simulink model "PubIfDecisionTOS_MDL"  (R2020b)
settings: configuration reference "DspaceConfig" (kept outside this file)
PostLoadFcn:
  | if any(exist('dsrtsu_mdlpostloadfcn', 'file') ~= 0), dsrtsu_mdlpostloadfcn('Execute', bdroot); end
InitFcn:
  | , if any(exist('dsmpb_private', 'file') ~= 0), dsmpb_private('dsmpb_mdlclblib', 'Init', bdroot); end,
undefined symbols (not defined in the file or in its folder): C_TOS_ACCEgoRAxletoFbumplength_m, C_TOS_ACCTargetFront_Flag, C_TOS_AEBJAPedObjDxThre_Val, C_TOS_AEBJAPedObjDyThre_Val, C_TOS_AEBJATargetSize_Val, C_TOS_AEBJAVehObjDxThre_Val, C_TOS_AEBJAVehObjDyThre_Val, C_TOS_AEBJuncPedTargetSize_Val, C_TOS_AEBLatObjDxThre_Val, C_TOS_AEBLatPedDyThre_Val, C_TOS_AEBLatTargetSize_Val, C_TOS_AEBLongTargetInEgoFront_Flag, C_TOS_axAbsGround_Parameter, C_TOS_CameraConfirmedFlag, C_TOS_CNsubjWidth, C_TOS_CurrentLaneCoreMinWidth_Val, C_TOS_CutInProb_Val_Zero, C_TOS_CutOutProb_Val_Zero, C_TOS_D2R_Val, C_TOS_DefaultValueObjectToCenterLine_dy, C_TOS_EgoCarWidth_Val, C_TOS_EgoDxRefPoint_m, C_TOS_EgoRAxletoFbumplength_m, C_TOS_HalfWidthVehicle_Con, C_TOS_HWA_CurrentLaneFlag, C_TOS_HWA_LeftLaneFlag, C_TOS_HWA_MovingDir_Vaild, C_TOS_HWA_MovState_Vaild, C_TOS_HWA_RightLaneFlag, C_TOS_LaneLineCourseErrorFront, C_TOS_LaneLineCourseErrorRear, C_TOS_MotorbikeDefaultWidth_m, C_TOS_NumberOfEffectiveTargets, C_TOS_Obj_Age_Val, C_TOS_Objdx_Constraint_Val, C_TOS_ObjectDefaultWidth_m, C_TOS_ObjInCurrentLane_Val, C_TOS_ObjInCurrentLaneValid, C_TOS_ObjInLeftLaneValid, C_TOS_ObjInRightLaneValid, C_TOS_ObjNotInCurrentLane_Val, C_TOS_ObjNotREElementType, C_TOS_ObjPredictDis_dy_ConstantVal_Zeros, C_TOS_ObjToCenterLine_ConstantVal_Zeros, C_TOS_OFMObjIDInvilad_Val, C_TOS_PIL_LatDisCons_Val_zero, C_TOS_PIL_ObjectCutInFlag_b, C_TOS_PIL_ObjectCutOutFlag_b, C_TOS_PIL_ObjLaneProb_al_Val, C_TOS_PP_ObjFusType_FC_Confirm_b, C_TOS_PP_ObjFusType_FC_FR_Confirm_b, C_TOS_PP_ObjFusType_FR_Confirm_b, C_TOS_RE_80BoolDefault_Val, C_TOS_RE_80Single181Default_Val, C_TOS_RE_80Single255Default_Val, C_TOS_RE_80Uint8Default_Val, C_TOS_RE_D2R, C_TOS_RE_D_180_Val, C_TOS_RE_InvalidObjectID_Val, C_TOS_RE_InvalidTargetChainDir_Val ... (+142)
libraries: simulink x1650, TOS_LIB x361, canfdmsglib x14
(part 20 of 69)

== system PubIfDecisionTOS_MDL/TOS_20201112/TOS_2012080320/TOS/ACC/TOS_ACCRightLane/ACC_Object_PreConfirm/ACC_Object_PreConfirm ==
  PP_ObjFusType_FC_FR_Confirm : Inport  Partition=on  PartitionDimension=1  PartitionWidth=1  PartitionOffset=0
  PP_ObjFusType_FR_Confirm : Inport  Port=2  Partition=on  PartitionDimension=1  PartitionWidth=1  PartitionOffset=0
  PP_ObjFusType_FC_Confirm : Inport  Port=3  Partition=on  PartitionDimension=1  PartitionWidth=1  PartitionOffset=0
  Object_ID : Inport  Port=4  OutDataTypeStr=uint8  Partition=on  PartitionDimension=1  PartitionWidth=1  PartitionOffset=0
  Obj_MovingState : Inport  Port=5  Partition=on  PartitionDimension=1  PartitionWidth=1  PartitionOffset=0
  Obj_Dx : Inport  Port=6  Partition=on  PartitionDimension=1  PartitionWidth=1  PartitionOffset=0
  Object_ObstacleProb : Inport  Port=7  Partition=on  PartitionDimension=1  PartitionWidth=1  PartitionOffset=0
  Object_DY : Inport  Port=8  Partition=on  PartitionDimension=1  PartitionWidth=1  PartitionOffset=0
  Object_ObjType : Inport  Port=9  Partition=on  PartitionDimension=1  PartitionWidth=1  PartitionOffset=0
  ACC_Target_ID_K1 : Inport  Port=10
  ACC_Target_Dx_K1 : Inport  Port=11
  ACC_Object_PreConfirm : Subsystem
  ACC_Object_PreConfirmDefault : Subsystem  TreatAsAtomicUnit=on
  Compare To Constant : simulink/Logic and Bit Operations/Compare To Constant  relop===  const=C_TOS_OFMObjIDInvilad_Val  OutDataTypeStr=boolean
      settings: AttributesFormatString=C_TOS_OFMObjIDInvilad_Val = 0
  For Each : ForEach  DisableCoverage=on
  If : If  IfExpression=u1 ~= 0
  Merge{,1,3..5} (5 alike) : Merge
  TOS_ACC_TargetPre_Confirm_FiltFlag : Outport  ConcatenationDimension=1
  TOS_ACC_TargetPre_FusionTypeFlag_ObserVale : Outport  Port=2  ConcatenationDimension=1
  TOS_ACC_TargetPre_PassedbyTarget_ObserVale : Outport  Port=3  ConcatenationDimension=1
  TOS_ACC_TargetPre_ObjType_ObserVale : Outport  Port=4  ConcatenationDimension=1
  TOS_ACC_DyConfirm_ObserVale : Outport  Port=5  ConcatenationDimension=1
  wires:
  Merge4/1 -> TOS_ACC_DyConfirm_ObserVale/1
  Merge3/1 -> TOS_ACC_TargetPre_ObjType_ObserVale/1
  Merge1/1 -> TOS_ACC_TargetPre_PassedbyTarget_ObserVale/1
  Merge5/1 -> TOS_ACC_TargetPre_FusionTypeFlag_ObserVale/1
  Merge/1 -> TOS_ACC_TargetPre_Confirm_FiltFlag/1
  ACC_Object_PreConfirmDefault/5(TOS_ACC_DyConfirm_ObserVale) -> Merge4/1
  ACC_Object_PreConfirmDefault/4(TOS_ACC_TargetPre_ObjType_ObserVale) -> Merge3/1
  ACC_Object_PreConfirmDefault/3(TOS_ACC_TargetPre_PassedbyTarget_ObserVale) -> Merge1/1
  ACC_Object_PreConfirmDefault/2(TOS_ACC_TargetPre_FusionTypeFlag_ObserVale) -> Merge5/1
  ACC_Object_PreConfirmDefault/1(TOS_ACC_TargetPre_Confirm_FiltFlag) -> Merge/1
  ACC_Object_PreConfirm/5(TOS_ACC_DyConfirm_ObserVale) -> Merge4/2
  ACC_Object_PreConfirm/4(TOS_ACC_TargetPre_ObjType_ObserVale) -> Merge3/2
  ACC_Object_PreConfirm/3(TOS_ACC_TargetPre_PassedbyTarget_ObserVale) -> Merge1/2
  ACC_Object_PreConfirm/2(TOS_ACC_TargetPre_FusionTypeFlag_ObserVale) -> Merge5/2
  ACC_Object_PreConfirm/1(TOS_ACC_TargetPre_Confirm_FiltFlag) -> Merge/2
  Object_ObjType/1 -> ACC_Object_PreConfirm/9(Object_ObjType)
  [Object_ID] -> ACC_Object_PreConfirm/1(Object_ID)
  ACC_Target_Dx_K1/1 -> ACC_Object_PreConfirm/11(ACC_Target_Dx_K1)
  ACC_Target_ID_K1/1 -> ACC_Object_PreConfirm/10(ACC_Target_ID_K1)
  Object_DY/1 -> ACC_Object_PreConfirm/8(Object_DY)
  Object_ObstacleProb/1 -> ACC_Object_PreConfirm/7(Object_ObstacleProb)
  Obj_Dx/1 -> ACC_Object_PreConfirm/6(Obj_Dx)
  Obj_MovingState/1 -> ACC_Object_PreConfirm/5(Obj_MovingState)
  PP_ObjFusType_FC_Confirm/1 -> ACC_Object_PreConfirm/4(PP_ObjFusType_FC_Confirm)
  If/2 -> ACC_Object_PreConfirm/Action
  If/1 -> ACC_Object_PreConfirmDefault/Action
  Object_ID/1 -> Compare To Constant/1, [Object_ID]
  Compare To Constant/1 -> If/1
  PP_ObjFusType_FR_Confirm/1 -> ACC_Object_PreConfirm/3(PP_ObjFusType_FR_Confirm)
  PP_ObjFusType_FC_FR_Confirm/1 -> ACC_Object_PreConfirm/2(PP_ObjFusType_FC_FR_Confirm)

== system PubIfDecisionTOS_MDL/TOS_20201112/TOS_2012080320/TOS/AEB/TOS_AEBJunct1105/AEBJunc_Object_Condition/AEBJA_TargetCondition ==
  Object_ID : Inport  OutDataTypeStr=uint8  Partition=on  PartitionDimension=1  PartitionWidth=1  PartitionOffset=0
  PP_ObjFusType_FC_FR_Confirm : Inport  Port=2  Partition=on  PartitionDimension=1  PartitionWidth=1  PartitionOffset=0
  PP_ObjFusType_FR_Confirm : Inport  Port=3  Partition=on  PartitionDimension=1  PartitionWidth=1  PartitionOffset=0
  ObjectType : Inport  Port=4  Partition=on  PartitionDimension=1  PartitionWidth=1  PartitionOffset=0
  Object_Dx : Inport  Port=5  Partition=on  PartitionDimension=1  PartitionWidth=1  PartitionOffset=0
  Object_Dy : Inport  Port=6  Partition=on  PartitionDimension=1  PartitionWidth=1  PartitionOffset=0
  PP_ObjMovingDirSignalProcessing : Inport  Port=7  Partition=on  PartitionDimension=1  PartitionWidth=1  PartitionOffset=0
  Object_HeadingAngle : Inport  Port=8  Partition=on  PartitionDimension=1  PartitionWidth=1  PartitionOffset=0
  Object_VX : Inport  Port=9  Partition=on  PartitionDimension=1  PartitionWidth=1  PartitionOffset=0
  Object_VY : Inport  Port=10  Partition=on  PartitionDimension=1  PartitionWidth=1  PartitionOffset=0
  VIE_EgoVelocity : Inport  Port=11
  psiDtOpt : Inport  Port=12
  axvRefMs2 : Inport  Port=13
  Object_MovingState : Inport  Port=14  Partition=on  PartitionDimension=1  PartitionWidth=1  PartitionOffset=0
  AEBJunc_Target_ObjectID_K1 : Inport  Port=15
  AEBJunc_Target_ObjectType_K1 : Inport  Port=16
  Compare To Constant : simulink/Logic and Bit Operations/Compare To Constant  relop===  const=C_TOS_OFMObjIDInvilad_Val  OutDataTypeStr=boolean
      settings: AttributesFormatString=C_TOS_OFMObjIDInvilad_Val = 0
  For Each : ForEach  DisableCoverage=on
  If : If  IfExpression=u1 ~= 0
  Merge{,1..10} (11 alike) : Merge
  TOS_AEBJunc_TargetsCondition : Subsystem
  TOS_AEBJunc_TargetsConditionDefault : Subsystem  TreatAsAtomicUnit=on
  TOS_AEBJunc_PedTargets_Dx : Outport  ConcatenationDimension=1
  TOS_AEBJunc_VehTargets_Dx : Outport  Port=2  ConcatenationDimension=1
  AEBJunc_PedTargetFusionType_observal : Outport  Port=3  ConcatenationDimension=1
  AEBJunc_PedTargetObjectType_observal : Outport  Port=4  ConcatenationDimension=1
  AEBJunc_PedTargetDXDY_observal : Outport  Port=5  ConcatenationDimension=1
  AEBJunc_PedTargetMovDir_observal : Outport  Port=6  ConcatenationDimension=1
  AEBJunc_VehTargetFusionType_observal : Outport  Port=7  ConcatenationDimension=1
  AEBJunc_VehTargetObjectType_observal : Outport  Port=8  ConcatenationDimension=1
  AEBJunc_VehTargetDXDY_observal : Outport  Port=9  ConcatenationDimension=1
  AEBJunc_VehTargetMovDir_observal : Outport  Port=10  ConcatenationDimension=1
  AEBJunc_VehTargetMovState_observal : Outport  Port=11  ConcatenationDimension=1
  wires:
  PP_ObjFusType_FC_FR_Confirm/1 -> TOS_AEBJunc_TargetsCondition/2(PP_ObjFusType_FC_FR_Confirm)
  PP_ObjFusType_FR_Confirm/1 -> TOS_AEBJunc_TargetsCondition/3(PP_ObjFusType_FR_Confirm)
  Object_VY/1 -> TOS_AEBJunc_TargetsCondition/10(Object_VY)
  VIE_EgoVelocity/1 -> TOS_AEBJunc_TargetsCondition/11(VIE_EgoVelocity)
  Object_VX/1 -> TOS_AEBJunc_TargetsCondition/9(Object_VX)
  PP_ObjMovingDirSignalProcessing/1 -> TOS_AEBJunc_TargetsCondition/7(PP_ObjMovingDirSignalProcessing)
  Object_HeadingAngle/1 -> TOS_AEBJunc_TargetsCondition/8(Object_HeadingAngle)
  ObjectType/1 -> TOS_AEBJunc_TargetsCondition/4(ObjectType)
  TOS_AEBJunc_TargetsConditionDefault/1(TOS_AEBJunc_PedTargetsDx) -> Merge/1
  If/2 -> TOS_AEBJunc_TargetsCondition/Action
  If/1 -> TOS_AEBJunc_TargetsConditionDefault/Action
  Object_ID/1 -> Compare To Constant/1, [Object_ID]
  Compare To Constant/1 -> If/1
  TOS_AEBJunc_TargetsCondition/1(TOS_AEBJunc_PedTargetsDx) -> Merge/2
  Object_Dy/1 -> TOS_AEBJunc_TargetsCondition/6(Object_Dy)
  Object_Dx/1 -> TOS_AEBJunc_TargetsCondition/5(Object_Dx)
  Merge/1 -> TOS_AEBJunc_PedTargets_Dx/1
  TOS_AEBJunc_TargetsCondition/3(AEBJunc_PedTargetFusionType_observal) -> Merge1/2
  TOS_AEBJunc_TargetsConditionDefault/3(AEBJunc_PedTargetFusionType_observal) -> Merge1/1
  TOS_AEBJunc_TargetsConditionDefault/4(AEBJunc_PedTargetObjectType_observal) -> Merge2/1
  TOS_AEBJunc_TargetsCondition/4(AEBJunc_PedTargetObjectType_observal) -> Merge2/2
  TOS_AEBJunc_TargetsCondition/5(AEBJunc_PedTargetDXDY_observal) -> Merge3/2
  TOS_AEBJunc_TargetsConditionDefault/5(AEBJunc_PedTargetDXDY_observal) -> Merge3/1
  TOS_AEBJunc_TargetsConditionDefault/6(AEBJunc_PedTargetMovDir_observal) -> Merge4/1
  TOS_AEBJunc_TargetsCondition/6(AEBJunc_PedTargetMovDir_observal) -> Merge4/2
  Merge1/1 -> AEBJunc_PedTargetFusionType_observal/1
  Merge2/1 -> AEBJunc_PedTargetObjectType_observal/1
  Merge3/1 -> AEBJunc_PedTargetDXDY_observal/1
  Merge4/1 -> AEBJunc_PedTargetMovDir_observal/1
  [Object_ID] -> TOS_AEBJunc_TargetsCondition/1(Object_ID)  "Object_ID"
  AEBJunc_Target_ObjectID_K1/1 -> TOS_AEBJunc_TargetsCondition/15(AEBJunc_Target_ObjectID_K1)
  psiDtOpt/1 -> TOS_AEBJunc_TargetsCondition/12(psiDtOpt)
  axvRefMs2/1 -> TOS_AEBJunc_TargetsCondition/13(axvRefMs2)  "axvRefMs2"
  AEBJunc_Target_ObjectType_K1/1 -> TOS_AEBJunc_TargetsCondition/16(AEBJunc_Target_ObjectType_K1)  "AEBJunc_Target_ObjectType_K1"
  Merge5/1 -> TOS_AEBJunc_VehTargets_Dx/1
  TOS_AEBJunc_TargetsCondition/2(TOS_AEBJunc_VehTargetsDx) -> Merge5/2
  TOS_AEBJunc_TargetsConditionDefault/2(TOS_AEBJunc_VehTargetsDx) -> Merge5/1
  Merge9/1 -> AEBJunc_VehTargetMovDir_observal/1
  Merge8/1 -> AEBJunc_VehTargetDXDY_observal/1
  Merge7/1 -> AEBJunc_VehTargetObjectType_observal/1
  Merge6/1 -> AEBJunc_VehTargetFusionType_observal/1
  TOS_AEBJunc_TargetsCondition/10(AEBJunc_VehTargetMovDir_observal) -> Merge9/2
  TOS_AEBJunc_TargetsConditionDefault/10(AEBJunc_VehTargetMovDir_observal) -> Merge9/1
  TOS_AEBJunc_TargetsConditionDefault/9(AEBJunc_VehTargetDXDY_observal) -> Merge8/1
  TOS_AEBJunc_TargetsCondition/9(AEBJunc_VehTargetDXDY_observal) -> Merge8/2
  TOS_AEBJunc_TargetsCondition/8(AEBJunc_VehTargetObjectType_observal) -> Merge7/2
  TOS_AEBJunc_TargetsConditionDefault/8(AEBJunc_VehTargetObjectType_observal) -> Merge7/1
  TOS_AEBJunc_TargetsConditionDefault/7(AEBJunc_VehTargetFusionType_observal) -> Merge6/1
  TOS_AEBJunc_TargetsCondition/7(AEBJunc_VehTargetFusionType_observal) -> Merge6/2
  Object_MovingState/1 -> TOS_AEBJunc_TargetsCondition/14(Object_MovingState)  "Object_MovingState"
  TOS_AEBJunc_TargetsConditionDefault/11(AEBJunc_VehTargetMovState_observal) -> Merge10/1
  TOS_AEBJunc_TargetsCondition/11(AEBJunc_VehTargetMovState_observal) -> Merge10/2
  Merge10/1 -> AEBJunc_VehTargetMovState_observal/1

== system PubIfDecisionTOS_MDL/TOS_20201112/TOS_2012080320/TOS/AEB/TOS_AEBJunct1105/AEBJunc_Object_Condition1/AEBJA_TargetCondition ==
  Object_ID : Inport  OutDataTypeStr=uint8  Partition=on  PartitionDimension=1  PartitionWidth=1  PartitionOffset=0
  PP_ObjFusType_FC_FR_Confirm : Inport  Port=2  Partition=on  PartitionDimension=1  PartitionWidth=1  PartitionOffset=0
  PP_ObjFusType_FR_Confirm : Inport  Port=3  Partition=on  PartitionDimension=1  PartitionWidth=1  PartitionOffset=0
  ObjectType : Inport  Port=4  Partition=on  PartitionDimension=1  PartitionWidth=1  PartitionOffset=0
  Object_Dx : Inport  Port=5  Partition=on  PartitionDimension=1  PartitionWidth=1  PartitionOffset=0
  Object_Dy : Inport  Port=6  Partition=on  PartitionDimension=1  PartitionWidth=1  PartitionOffset=0
  PP_ObjMovingDirSignalProcessing : Inport  Port=7  Partition=on  PartitionDimension=1  PartitionWidth=1  PartitionOffset=0
  Object_HeadingAngle : Inport  Port=8  Partition=on  PartitionDimension=1  PartitionWidth=1  PartitionOffset=0
  Object_VX : Inport  Port=9  Partition=on  PartitionDimension=1  PartitionWidth=1  PartitionOffset=0
  Object_VY : Inport  Port=10  Partition=on  PartitionDimension=1  PartitionWidth=1  PartitionOffset=0
  VIE_EgoVelocity : Inport  Port=11
  psiDtOpt : Inport  Port=12
  axvRefMs2 : Inport  Port=13
  Object_MovingState : Inport  Port=14  Partition=on  PartitionDimension=1  PartitionWidth=1  PartitionOffset=0
  AEBJunc_Target_ObjectID_K1 : Inport  Port=15
  AEBJunc_Target_ObjectType_K1 : Inport  Port=16
  Compare To Constant : simulink/Logic and Bit Operations/Compare To Constant  relop===  const=C_TOS_OFMObjIDInvilad_Val  OutDataTypeStr=boolean
      settings: AttributesFormatString=C_TOS_OFMObjIDInvilad_Val = 0
  For Each : ForEach  DisableCoverage=on
  If : If  IfExpression=u1 ~= 0
  Merge{,1..10} (11 alike) : Merge
  TOS_AEBJunc_TargetsCondition : Subsystem
  TOS_AEBJunc_TargetsConditionDefault : Subsystem  TreatAsAtomicUnit=on
  TOS_AEBJunc_PedTargets_Dx : Outport  ConcatenationDimension=1
  TOS_AEBJunc_VehTargets_Dx : Outport  Port=2  ConcatenationDimension=1
  AEBJunc_PedTargetFusionType_observal : Outport  Port=3  ConcatenationDimension=1
  AEBJunc_PedTargetObjectType_observal : Outport  Port=4  ConcatenationDimension=1
  AEBJunc_PedTargetDXDY_observal : Outport  Port=5  ConcatenationDimension=1
  AEBJunc_PedTargetMovDir_observal : Outport  Port=6  ConcatenationDimension=1
  AEBJunc_VehTargetFusionType_observal : Outport  Port=7  ConcatenationDimension=1
  AEBJunc_VehTargetObjectType_observal : Outport  Port=8  ConcatenationDimension=1
  AEBJunc_VehTargetDXDY_observal : Outport  Port=9  ConcatenationDimension=1
  AEBJunc_VehTargetMovDir_observal : Outport  Port=10  ConcatenationDimension=1
  AEBJunc_VehTargetMovState_observal : Outport  Port=11  ConcatenationDimension=1
  wires:
  Merge10/1 -> AEBJunc_VehTargetMovState_observal/1
  TOS_AEBJunc_TargetsCondition/11(AEBJunc_VehTargetMovState_observal) -> Merge10/2
  TOS_AEBJunc_TargetsConditionDefault/11(AEBJunc_VehTargetMovState_observal) -> Merge10/1
  Object_MovingState/1 -> TOS_AEBJunc_TargetsCondition/14(Object_MovingState)  "Object_MovingState"
  TOS_AEBJunc_TargetsCondition/7(AEBJunc_VehTargetFusionType_observal) -> Merge6/2
  TOS_AEBJunc_TargetsConditionDefault/7(AEBJunc_VehTargetFusionType_observal) -> Merge6/1
  TOS_AEBJunc_TargetsConditionDefault/8(AEBJunc_VehTargetObjectType_observal) -> Merge7/1
  TOS_AEBJunc_TargetsCondition/8(AEBJunc_VehTargetObjectType_observal) -> Merge7/2
  TOS_AEBJunc_TargetsCondition/9(AEBJunc_VehTargetDXDY_observal) -> Merge8/2
  TOS_AEBJunc_TargetsConditionDefault/9(AEBJunc_VehTargetDXDY_observal) -> Merge8/1
  TOS_AEBJunc_TargetsConditionDefault/10(AEBJunc_VehTargetMovDir_observal) -> Merge9/1
  TOS_AEBJunc_TargetsCondition/10(AEBJunc_VehTargetMovDir_observal) -> Merge9/2
  Merge6/1 -> AEBJunc_VehTargetFusionType_observal/1
  Merge7/1 -> AEBJunc_VehTargetObjectType_observal/1
  Merge8/1 -> AEBJunc_VehTargetDXDY_observal/1
  Merge9/1 -> AEBJunc_VehTargetMovDir_observal/1
  TOS_AEBJunc_TargetsConditionDefault/2(TOS_AEBJunc_VehTargetsDx) -> Merge5/1
  TOS_AEBJunc_TargetsCondition/2(TOS_AEBJunc_VehTargetsDx) -> Merge5/2
  Merge5/1 -> TOS_AEBJunc_VehTargets_Dx/1
  AEBJunc_Target_ObjectType_K1/1 -> TOS_AEBJunc_TargetsCondition/16(AEBJunc_Target_ObjectType_K1)  "AEBJunc_Target_ObjectType_K1"
  axvRefMs2/1 -> TOS_AEBJunc_TargetsCondition/13(axvRefMs2)  "axvRefMs2"
  psiDtOpt/1 -> TOS_AEBJunc_TargetsCondition/12(psiDtOpt)
  AEBJunc_Target_ObjectID_K1/1 -> TOS_AEBJunc_TargetsCondition/15(AEBJunc_Target_ObjectID_K1)
  [Object_ID] -> TOS_AEBJunc_TargetsCondition/1(Object_ID)  "Object_ID"
  Merge4/1 -> AEBJunc_PedTargetMovDir_observal/1
  Merge3/1 -> AEBJunc_PedTargetDXDY_observal/1
  Merge2/1 -> AEBJunc_PedTargetObjectType_observal/1
  Merge1/1 -> AEBJunc_PedTargetFusionType_observal/1
  TOS_AEBJunc_TargetsCondition/6(AEBJunc_PedTargetMovDir_observal) -> Merge4/2
  TOS_AEBJunc_TargetsConditionDefault/6(AEBJunc_PedTargetMovDir_observal) -> Merge4/1
  TOS_AEBJunc_TargetsConditionDefault/5(AEBJunc_PedTargetDXDY_observal) -> Merge3/1
  TOS_AEBJunc_TargetsCondition/5(AEBJunc_PedTargetDXDY_observal) -> Merge3/2
  TOS_AEBJunc_TargetsCondition/4(AEBJunc_PedTargetObjectType_observal) -> Merge2/2
  TOS_AEBJunc_TargetsConditionDefault/4(AEBJunc_PedTargetObjectType_observal) -> Merge2/1
  TOS_AEBJunc_TargetsConditionDefault/3(AEBJunc_PedTargetFusionType_observal) -> Merge1/1
  TOS_AEBJunc_TargetsCondition/3(AEBJunc_PedTargetFusionType_observal) -> Merge1/2
  Merge/1 -> TOS_AEBJunc_PedTargets_Dx/1
  Object_Dx/1 -> TOS_AEBJunc_TargetsCondition/5(Object_Dx)
  Object_Dy/1 -> TOS_AEBJunc_TargetsCondition/6(Object_Dy)
  TOS_AEBJunc_TargetsCondition/1(TOS_AEBJunc_PedTargetsDx) -> Merge/2
  Compare To Constant/1 -> If/1
  Object_ID/1 -> [Object_ID], Compare To Constant/1
  If/1 -> TOS_AEBJunc_TargetsConditionDefault/Action
  If/2 -> TOS_AEBJunc_TargetsCondition/Action
  TOS_AEBJunc_TargetsConditionDefault/1(TOS_AEBJunc_PedTargetsDx) -> Merge/1
  ObjectType/1 -> TOS_AEBJunc_TargetsCondition/4(ObjectType)
  Object_HeadingAngle/1 -> TOS_AEBJunc_TargetsCondition/8(Object_HeadingAngle)
  PP_ObjMovingDirSignalProcessing/1 -> TOS_AEBJunc_TargetsCondition/7(PP_ObjMovingDirSignalProcessing)
  Object_VX/1 -> TOS_AEBJunc_TargetsCondition/9(Object_VX)
  VIE_EgoVelocity/1 -> TOS_AEBJunc_TargetsCondition/11(VIE_EgoVelocity)
  Object_VY/1 -> TOS_AEBJunc_TargetsCondition/10(Object_VY)
  PP_ObjFusType_FR_Confirm/1 -> TOS_AEBJunc_TargetsCondition/3(PP_ObjFusType_FR_Confirm)
  PP_ObjFusType_FC_FR_Confirm/1 -> TOS_AEBJunc_TargetsCondition/2(PP_ObjFusType_FC_FR_Confirm)

== system PubIfDecisionTOS_MDL/TOS_20201112/TOS_2012080320/TOS/AEB/TOS_AEBJunct1105/AEBJunctionTargetInfor/AEBJuncTargetObjectType ==
  OFM_SignalVerification : Inport
  AEBJunc_Target_ObjectID_K1 : Inport  Port=2
  AEBJunc_Target_ObjectType_K1 : Inport  Port=3
  TOS_AEBJuncTrg_Index : Inport  Port=4  OutDataTypeStr=uint8  Partition=on  PartitionDimension=1  PartitionWidth=1  PartitionOffset=0
  AEBJuncTargetObjectType : Subsystem  TreatAsAtomicUnit=on
  AEBJuncTargetObjectTypeDefault : Subsystem  TreatAsAtomicUnit=on
  Compare To Constant1 : simulink/Logic and Bit Operations/Compare To Constant  relop===  const=C_TOS_OFMObjIDInvilad_Val  OutDataTypeStr=boolean
      settings: AttributesFormatString=C_TOS_OFMObjIDInvilad_Val = 0
  For Each : ForEach  DisableCoverage=on
  If : If  IfExpression=u1
  Merge : Merge
  TOS_AEBJuncTargetObjectType : Outport  ConcatenationDimension=1
  wires:
  Merge/1 -> TOS_AEBJuncTargetObjectType/1
  AEBJuncTargetObjectTypeDefault/1(TOS_AEBJuncTargetObjectType) -> Merge/1
  AEBJuncTargetObjectType/1(AEBLat_TargetObjectType) -> Merge/2
  If/2 -> AEBJuncTargetObjectType/Action
  If/1 -> AEBJuncTargetObjectTypeDefault/Action
  OFM_SignalVerification/1 -> AEBJuncTargetObjectType/2(OFM_SignalVerification)
  Compare To Constant1/1 -> If/1
  TOS_AEBJuncTrg_Index/1 -> AEBJuncTargetObjectType/1(TOS_AEBJuncTrg_Index), Compare To Constant1/1
  AEBJunc_Target_ObjectID_K1/1 -> AEBJuncTargetObjectType/3(AEBJunc_Target_ObjectID_K1)  "AEBJunc_Target_ObjectID_K1"
  AEBJunc_Target_ObjectType_K1/1 -> AEBJuncTargetObjectType/4(AEBJunc_Target_ObjectType_K1)  "AEBJunc_Target_ObjectType_K1"

== system PubIfDecisionTOS_MDL/TOS_20201112/TOS_2012080320/TOS/AEB/TOS_AEBJunct_20201208/AEBJunc_Object_Condition/AEBJA_TargetCondition ==
  Object_ID : Inport  OutDataTypeStr=uint8  Partition=on  PartitionDimension=1  PartitionWidth=1  PartitionOffset=0
  PP_ObjFusType_FC_FR_Confirm : Inport  Port=2  Partition=on  PartitionDimension=1  PartitionWidth=1  PartitionOffset=0
  PP_ObjFusType_FR_Confirm : Inport  Port=3  Partition=on  PartitionDimension=1  PartitionWidth=1  PartitionOffset=0
  ObjectType : Inport  Port=4  Partition=on  PartitionDimension=1  PartitionWidth=1  PartitionOffset=0
  Object_Dx : Inport  Port=5  Partition=on  PartitionDimension=1  PartitionWidth=1  PartitionOffset=0
  Object_Dy : Inport  Port=6  Partition=on  PartitionDimension=1  PartitionWidth=1  PartitionOffset=0
  PP_ObjMovingDirSignalProcessing : Inport  Port=7  Partition=on  PartitionDimension=1  PartitionWidth=1  PartitionOffset=0
  Object_HeadingAngle : Inport  Port=8  Partition=on  PartitionDimension=1  PartitionWidth=1  PartitionOffset=0
  Object_VX : Inport  Port=9  Partition=on  PartitionDimension=1  PartitionWidth=1  PartitionOffset=0
  Object_VY : Inport  Port=10  Partition=on  PartitionDimension=1  PartitionWidth=1  PartitionOffset=0
  VIE_EgoVelocity : Inport  Port=11
  psiDtOpt : Inport  Port=12
  axvRefMs2 : Inport  Port=13
  Object_MovingState : Inport  Port=14  Partition=on  PartitionDimension=1  PartitionWidth=1  PartitionOffset=0
  AEBJunc_Target_ObjectID_K1 : Inport  Port=15
  AEBJunc_Target_ObjectType_K1 : Inport  Port=16
  Compare To Constant : simulink/Logic and Bit Operations/Compare To Constant  relop===  const=C_TOS_OFMObjIDInvilad_Val  OutDataTypeStr=boolean
      settings: AttributesFormatString=C_TOS_OFMObjIDInvilad_Val = 0
  For Each : ForEach  DisableCoverage=on
  If : If  IfExpression=u1 ~= 0
  Merge{,1..10} (11 alike) : Merge
  TOS_AEBJunc_TargetsCondition : Subsystem
  TOS_AEBJunc_TargetsConditionDefault : Subsystem  TreatAsAtomicUnit=on
  TOS_AEBJunc_PedTargets_Dx : Outport  ConcatenationDimension=1
  TOS_AEBJunc_VehTargets_Dx : Outport  Port=2  ConcatenationDimension=1
  AEBJunc_PedTargetFusionType_observal : Outport  Port=3  ConcatenationDimension=1
  AEBJunc_PedTargetObjectType_observal : Outport  Port=4  ConcatenationDimension=1
  AEBJunc_PedTargetDXDY_observal : Outport  Port=5  ConcatenationDimension=1
  AEBJunc_PedTargetMovDir_observal : Outport  Port=6  ConcatenationDimension=1
  AEBJunc_VehTargetFusionType_observal : Outport  Port=7  ConcatenationDimension=1
  AEBJunc_VehTargetObjectType_observal : Outport  Port=8  ConcatenationDimension=1
  AEBJunc_VehTargetDXDY_observal : Outport  Port=9  ConcatenationDimension=1
  AEBJunc_VehTargetMovDir_observal : Outport  Port=10  ConcatenationDimension=1
  AEBJunc_VehTargetMovState_observal : Outport  Port=11  ConcatenationDimension=1
  wires:
  PP_ObjFusType_FC_FR_Confirm/1 -> TOS_AEBJunc_TargetsCondition/2(PP_ObjFusType_FC_FR_Confirm)
  PP_ObjFusType_FR_Confirm/1 -> TOS_AEBJunc_TargetsCondition/3(PP_ObjFusType_FR_Confirm)
  Object_VY/1 -> TOS_AEBJunc_TargetsCondition/10(Object_VY)
  VIE_EgoVelocity/1 -> TOS_AEBJunc_TargetsCondition/11(VIE_EgoVelocity)
  Object_VX/1 -> TOS_AEBJunc_TargetsCondition/9(Object_VX)
  PP_ObjMovingDirSignalProcessing/1 -> TOS_AEBJunc_TargetsCondition/7(PP_ObjMovingDirSignalProcessing)
  Object_HeadingAngle/1 -> TOS_AEBJunc_TargetsCondition/8(Object_HeadingAngle)
  ObjectType/1 -> TOS_AEBJunc_TargetsCondition/4(ObjectType)
  TOS_AEBJunc_TargetsConditionDefault/1(TOS_AEBJunc_PedTargetsDx) -> Merge/1
  If/2 -> TOS_AEBJunc_TargetsCondition/Action
  If/1 -> TOS_AEBJunc_TargetsConditionDefault/Action
  Object_ID/1 -> Compare To Constant/1, [Object_ID]
  Compare To Constant/1 -> If/1
  TOS_AEBJunc_TargetsCondition/1(TOS_AEBJunc_PedTargetsDx) -> Merge/2
  Object_Dy/1 -> TOS_AEBJunc_TargetsCondition/6(Object_Dy)
  Object_Dx/1 -> TOS_AEBJunc_TargetsCondition/5(Object_Dx)
  Merge/1 -> TOS_AEBJunc_PedTargets_Dx/1
  TOS_AEBJunc_TargetsCondition/3(AEBJunc_PedTargetFusionType_observal) -> Merge1/2
  TOS_AEBJunc_TargetsConditionDefault/3(AEBJunc_PedTargetFusionType_observal) -> Merge1/1
  TOS_AEBJunc_TargetsConditionDefault/4(AEBJunc_PedTargetObjectType_observal) -> Merge2/1
  TOS_AEBJunc_TargetsCondition/4(AEBJunc_PedTargetObjectType_observal) -> Merge2/2
  TOS_AEBJunc_TargetsCondition/5(AEBJunc_PedTargetDXDY_observal) -> Merge3/2
  TOS_AEBJunc_TargetsConditionDefault/5(AEBJunc_PedTargetDXDY_observal) -> Merge3/1
  TOS_AEBJunc_TargetsConditionDefault/6(AEBJunc_PedTargetMovDir_observal) -> Merge4/1
  TOS_AEBJunc_TargetsCondition/6(AEBJunc_PedTargetMovDir_observal) -> Merge4/2
  Merge1/1 -> AEBJunc_PedTargetFusionType_observal/1
  Merge2/1 -> AEBJunc_PedTargetObjectType_observal/1
  Merge3/1 -> AEBJunc_PedTargetDXDY_observal/1
  Merge4/1 -> AEBJunc_PedTargetMovDir_observal/1
  [Object_ID] -> TOS_AEBJunc_TargetsCondition/1(Object_ID)  "Object_ID"
  AEBJunc_Target_ObjectID_K1/1 -> TOS_AEBJunc_TargetsCondition/15(AEBJunc_Target_ObjectID_K1)
  psiDtOpt/1 -> TOS_AEBJunc_TargetsCondition/12(psiDtOpt)
  axvRefMs2/1 -> TOS_AEBJunc_TargetsCondition/13(axvRefMs2)  "axvRefMs2"
  AEBJunc_Target_ObjectType_K1/1 -> TOS_AEBJunc_TargetsCondition/16(AEBJunc_Target_ObjectType_K1)  "AEBJunc_Target_ObjectType_K1"
  Merge5/1 -> TOS_AEBJunc_VehTargets_Dx/1
  TOS_AEBJunc_TargetsCondition/2(TOS_AEBJunc_VehTargetsDx) -> Merge5/2
  TOS_AEBJunc_TargetsConditionDefault/2(TOS_AEBJunc_VehTargetsDx) -> Merge5/1
  Merge9/1 -> AEBJunc_VehTargetMovDir_observal/1
  Merge8/1 -> AEBJunc_VehTargetDXDY_observal/1
  Merge7/1 -> AEBJunc_VehTargetObjectType_observal/1
  Merge6/1 -> AEBJunc_VehTargetFusionType_observal/1
  TOS_AEBJunc_TargetsCondition/10(AEBJunc_VehTargetMovDir_observal) -> Merge9/2
  TOS_AEBJunc_TargetsConditionDefault/10(AEBJunc_VehTargetMovDir_observal) -> Merge9/1
  TOS_AEBJunc_TargetsConditionDefault/9(AEBJunc_VehTargetDXDY_observal) -> Merge8/1
  TOS_AEBJunc_TargetsCondition/9(AEBJunc_VehTargetDXDY_observal) -> Merge8/2
  TOS_AEBJunc_TargetsCondition/8(AEBJunc_VehTargetObjectType_observal) -> Merge7/2
  TOS_AEBJunc_TargetsConditionDefault/8(AEBJunc_VehTargetObjectType_observal) -> Merge7/1
  TOS_AEBJunc_TargetsConditionDefault/7(AEBJunc_VehTargetFusionType_observal) -> Merge6/1
  TOS_AEBJunc_TargetsCondition/7(AEBJunc_VehTargetFusionType_observal) -> Merge6/2
  Object_MovingState/1 -> TOS_AEBJunc_TargetsCondition/14(Object_MovingState)  "Object_MovingState"
  TOS_AEBJunc_TargetsConditionDefault/11(AEBJunc_VehTargetMovState_observal) -> Merge10/1
  TOS_AEBJunc_TargetsCondition/11(AEBJunc_VehTargetMovState_observal) -> Merge10/2
  Merge10/1 -> AEBJunc_VehTargetMovState_observal/1

== system PubIfDecisionTOS_MDL/TOS_20201112/TOS_2012080320/TOS/AEB/TOS_AEBJunct_20201208/AEBJunc_Object_Condition1/AEBJA_TargetCondition ==
  Object_ID : Inport  OutDataTypeStr=uint8  Partition=on  PartitionDimension=1  PartitionWidth=1  PartitionOffset=0
  PP_ObjFusType_FC_FR_Confirm : Inport  Port=2  Partition=on  PartitionDimension=1  PartitionWidth=1  PartitionOffset=0
  PP_ObjFusType_FR_Confirm : Inport  Port=3  Partition=on  PartitionDimension=1  PartitionWidth=1  PartitionOffset=0
  ObjectType : Inport  Port=4  Partition=on  PartitionDimension=1  PartitionWidth=1  PartitionOffset=0
  Object_Dx : Inport  Port=5  Partition=on  PartitionDimension=1  PartitionWidth=1  PartitionOffset=0
  Object_Dy : Inport  Port=6  Partition=on  PartitionDimension=1  PartitionWidth=1  PartitionOffset=0
  PP_ObjMovingDirSignalProcessing : Inport  Port=7  Partition=on  PartitionDimension=1  PartitionWidth=1  PartitionOffset=0
  Object_HeadingAngle : Inport  Port=8  Partition=on  PartitionDimension=1  PartitionWidth=1  PartitionOffset=0
  Object_VX : Inport  Port=9  Partition=on  PartitionDimension=1  PartitionWidth=1  PartitionOffset=0
  Object_VY : Inport  Port=10  Partition=on  PartitionDimension=1  PartitionWidth=1  PartitionOffset=0
  VIE_EgoVelocity : Inport  Port=11
  psiDtOpt : Inport  Port=12
  axvRefMs2 : Inport  Port=13
  Object_MovingState : Inport  Port=14  Partition=on  PartitionDimension=1  PartitionWidth=1  PartitionOffset=0
  AEBJunc_Target_ObjectID_K1 : Inport  Port=15
  AEBJunc_Target_ObjectType_K1 : Inport  Port=16
  Compare To Constant : simulink/Logic and Bit Operations/Compare To Constant  relop===  const=C_TOS_OFMObjIDInvilad_Val  OutDataTypeStr=boolean
      settings: AttributesFormatString=C_TOS_OFMObjIDInvilad_Val = 0
  For Each : ForEach  DisableCoverage=on
  If : If  IfExpression=u1 ~= 0
  Merge{,1..10} (11 alike) : Merge
  TOS_AEBJunc_TargetsCondition : Subsystem
  TOS_AEBJunc_TargetsConditionDefault : Subsystem  TreatAsAtomicUnit=on
  TOS_AEBJunc_PedTargets_Dx : Outport  ConcatenationDimension=1
  TOS_AEBJunc_VehTargets_Dx : Outport  Port=2  ConcatenationDimension=1
  AEBJunc_PedTargetFusionType_observal : Outport  Port=3  ConcatenationDimension=1
  AEBJunc_PedTargetObjectType_observal : Outport  Port=4  ConcatenationDimension=1
  AEBJunc_PedTargetDXDY_observal : Outport  Port=5  ConcatenationDimension=1
  AEBJunc_PedTargetMovDir_observal : Outport  Port=6  ConcatenationDimension=1
  AEBJunc_VehTargetFusionType_observal : Outport  Port=7  ConcatenationDimension=1
  AEBJunc_VehTargetObjectType_observal : Outport  Port=8  ConcatenationDimension=1
  AEBJunc_VehTargetDXDY_observal : Outport  Port=9  ConcatenationDimension=1
  AEBJunc_VehTargetMovDir_observal : Outport  Port=10  ConcatenationDimension=1
  AEBJunc_VehTargetMovState_observal : Outport  Port=11  ConcatenationDimension=1
  wires:
  Merge10/1 -> AEBJunc_VehTargetMovState_observal/1
  TOS_AEBJunc_TargetsCondition/11(AEBJunc_VehTargetMovState_observal) -> Merge10/2
  TOS_AEBJunc_TargetsConditionDefault/11(AEBJunc_VehTargetMovState_observal) -> Merge10/1
  Object_MovingState/1 -> TOS_AEBJunc_TargetsCondition/14(Object_MovingState)  "Object_MovingState"
  TOS_AEBJunc_TargetsCondition/7(AEBJunc_VehTargetFusionType_observal) -> Merge6/2
  TOS_AEBJunc_TargetsConditionDefault/7(AEBJunc_VehTargetFusionType_observal) -> Merge6/1
  TOS_AEBJunc_TargetsConditionDefault/8(AEBJunc_VehTargetObjectType_observal) -> Merge7/1
  TOS_AEBJunc_TargetsCondition/8(AEBJunc_VehTargetObjectType_observal) -> Merge7/2
  TOS_AEBJunc_TargetsCondition/9(AEBJunc_VehTargetDXDY_observal) -> Merge8/2
  TOS_AEBJunc_TargetsConditionDefault/9(AEBJunc_VehTargetDXDY_observal) -> Merge8/1
  TOS_AEBJunc_TargetsConditionDefault/10(AEBJunc_VehTargetMovDir_observal) -> Merge9/1
  TOS_AEBJunc_TargetsCondition/10(AEBJunc_VehTargetMovDir_observal) -> Merge9/2
  Merge6/1 -> AEBJunc_VehTargetFusionType_observal/1
  Merge7/1 -> AEBJunc_VehTargetObjectType_observal/1
  Merge8/1 -> AEBJunc_VehTargetDXDY_observal/1
  Merge9/1 -> AEBJunc_VehTargetMovDir_observal/1
  TOS_AEBJunc_TargetsConditionDefault/2(TOS_AEBJunc_VehTargetsDx) -> Merge5/1
  TOS_AEBJunc_TargetsCondition/2(TOS_AEBJunc_VehTargetsDx) -> Merge5/2
  Merge5/1 -> TOS_AEBJunc_VehTargets_Dx/1
  AEBJunc_Target_ObjectType_K1/1 -> TOS_AEBJunc_TargetsCondition/16(AEBJunc_Target_ObjectType_K1)  "AEBJunc_Target_ObjectType_K1"
  axvRefMs2/1 -> TOS_AEBJunc_TargetsCondition/13(axvRefMs2)  "axvRefMs2"
  psiDtOpt/1 -> TOS_AEBJunc_TargetsCondition/12(psiDtOpt)
  AEBJunc_Target_ObjectID_K1/1 -> TOS_AEBJunc_TargetsCondition/15(AEBJunc_Target_ObjectID_K1)
  [Object_ID] -> TOS_AEBJunc_TargetsCondition/1(Object_ID)  "Object_ID"
  Merge4/1 -> AEBJunc_PedTargetMovDir_observal/1
  Merge3/1 -> AEBJunc_PedTargetDXDY_observal/1
  Merge2/1 -> AEBJunc_PedTargetObjectType_observal/1
  Merge1/1 -> AEBJunc_PedTargetFusionType_observal/1
  TOS_AEBJunc_TargetsCondition/6(AEBJunc_PedTargetMovDir_observal) -> Merge4/2
  TOS_AEBJunc_TargetsConditionDefault/6(AEBJunc_PedTargetMovDir_observal) -> Merge4/1
  TOS_AEBJunc_TargetsConditionDefault/5(AEBJunc_PedTargetDXDY_observal) -> Merge3/1
  TOS_AEBJunc_TargetsCondition/5(AEBJunc_PedTargetDXDY_observal) -> Merge3/2
  TOS_AEBJunc_TargetsCondition/4(AEBJunc_PedTargetObjectType_observal) -> Merge2/2
  TOS_AEBJunc_TargetsConditionDefault/4(AEBJunc_PedTargetObjectType_observal) -> Merge2/1
  TOS_AEBJunc_TargetsConditionDefault/3(AEBJunc_PedTargetFusionType_observal) -> Merge1/1
  TOS_AEBJunc_TargetsCondition/3(AEBJunc_PedTargetFusionType_observal) -> Merge1/2
  Merge/1 -> TOS_AEBJunc_PedTargets_Dx/1
  Object_Dx/1 -> TOS_AEBJunc_TargetsCondition/5(Object_Dx)
  Object_Dy/1 -> TOS_AEBJunc_TargetsCondition/6(Object_Dy)
  TOS_AEBJunc_TargetsCondition/1(TOS_AEBJunc_PedTargetsDx) -> Merge/2
  Compare To Constant/1 -> If/1
  Object_ID/1 -> [Object_ID], Compare To Constant/1
  If/1 -> TOS_AEBJunc_TargetsConditionDefault/Action
  If/2 -> TOS_AEBJunc_TargetsCondition/Action
  TOS_AEBJunc_TargetsConditionDefault/1(TOS_AEBJunc_PedTargetsDx) -> Merge/1
  ObjectType/1 -> TOS_AEBJunc_TargetsCondition/4(ObjectType)
  Object_HeadingAngle/1 -> TOS_AEBJunc_TargetsCondition/8(Object_HeadingAngle)
  PP_ObjMovingDirSignalProcessing/1 -> TOS_AEBJunc_TargetsCondition/7(PP_ObjMovingDirSignalProcessing)
  Object_VX/1 -> TOS_AEBJunc_TargetsCondition/9(Object_VX)
  VIE_EgoVelocity/1 -> TOS_AEBJunc_TargetsCondition/11(VIE_EgoVelocity)
  Object_VY/1 -> TOS_AEBJunc_TargetsCondition/10(Object_VY)
  PP_ObjFusType_FR_Confirm/1 -> TOS_AEBJunc_TargetsCondition/3(PP_ObjFusType_FR_Confirm)
  PP_ObjFusType_FC_FR_Confirm/1 -> TOS_AEBJunc_TargetsCondition/2(PP_ObjFusType_FC_FR_Confirm)

== system PubIfDecisionTOS_MDL/TOS_20201112/TOS_2012080320/TOS/AEB/TOS_AEBJunct_20201208/AEBJunctionTargetInfor/AEBJuncTargetObjectType ==
  OFM_SignalVerification : Inport
  AEBJunc_Target_ObjectID_K1 : Inport  Port=2
  AEBJunc_Target_ObjectType_K1 : Inport  Port=3
  TOS_AEBJuncTrg_Index : Inport  Port=4  OutDataTypeStr=uint8  Partition=on  PartitionDimension=1  PartitionWidth=1  PartitionOffset=0
  AEBJuncTargetObjectType : Subsystem  TreatAsAtomicUnit=on
  AEBJuncTargetObjectTypeDefault : Subsystem  TreatAsAtomicUnit=on
  Compare To Constant1 : simulink/Logic and Bit Operations/Compare To Constant  relop===  const=C_TOS_OFMObjIDInvilad_Val  OutDataTypeStr=boolean
      settings: AttributesFormatString=C_TOS_OFMObjIDInvilad_Val = 0
  For Each : ForEach  DisableCoverage=on
  If : If  IfExpression=u1
  Merge : Merge
  TOS_AEBJuncTargetObjectType : Outport  ConcatenationDimension=1
  wires:
  Merge/1 -> TOS_AEBJuncTargetObjectType/1
  AEBJuncTargetObjectTypeDefault/1(TOS_AEBJuncTargetObjectType) -> Merge/1
  AEBJuncTargetObjectType/1(AEBLat_TargetObjectType) -> Merge/2
  If/2 -> AEBJuncTargetObjectType/Action
  If/1 -> AEBJuncTargetObjectTypeDefault/Action
  OFM_SignalVerification/1 -> AEBJuncTargetObjectType/2(OFM_SignalVerification)
  Compare To Constant1/1 -> If/1
  TOS_AEBJuncTrg_Index/1 -> AEBJuncTargetObjectType/1(TOS_AEBJuncTrg_Index), Compare To Constant1/1
  AEBJunc_Target_ObjectID_K1/1 -> AEBJuncTargetObjectType/3(AEBJunc_Target_ObjectID_K1)  "AEBJunc_Target_ObjectID_K1"
  AEBJunc_Target_ObjectType_K1/1 -> AEBJuncTargetObjectType/4(AEBJunc_Target_ObjectType_K1)  "AEBJunc_Target_ObjectType_K1"

== system PubIfDecisionTOS_MDL/TOS_20201112/TOS_2012080320/TOS/AEB/TOS_AEBLatCro1105/AEBLatTrgInfor/AEBLatTargetObjectType ==
  OFM_SignalVerification : Inport
  AEBLat_Target_ObjectID_K1 : Inport  Port=2
  AEBLat_Target_ObjectType_K1 : Inport  Port=3
  TOS_AEBLatTrg_Index : Inport  Port=4  OutDataTypeStr=uint8  Partition=on  PartitionDimension=1  PartitionWidth=1  PartitionOffset=0
  AEBLatTargetObjectType : Subsystem  TreatAsAtomicUnit=on
  AEBLatTargetObjectTypeDefault : Subsystem  TreatAsAtomicUnit=on
  Compare To Constant1 : simulink/Logic and Bit Operations/Compare To Constant  relop===  const=C_TOS_OFMObjIDInvilad_Val  OutDataTypeStr=boolean
      settings: AttributesFormatString=C_TOS_OFMObjIDInvilad_Val = 0
  For Each : ForEach  DisableCoverage=on
  If : If  IfExpression=u1
  Merge : Merge
  TOS_AEBLatTargetObjectType : Outport  ConcatenationDimension=1
  wires:
  Merge/1 -> TOS_AEBLatTargetObjectType/1
  AEBLatTargetObjectTypeDefault/1(TOS_AEBLatTargetObjectType) -> Merge/1
  AEBLatTargetObjectType/1(AEBLat_TargetObjectType) -> Merge/2
  If/2 -> AEBLatTargetObjectType/Action
  If/1 -> AEBLatTargetObjectTypeDefault/Action
  OFM_SignalVerification/1 -> AEBLatTargetObjectType/2(OFM_SignalVerification)
  Compare To Constant1/1 -> If/1
  TOS_AEBLatTrg_Index/1 -> AEBLatTargetObjectType/1(TOS_AEBLatTrg_Index), Compare To Constant1/1
  AEBLat_Target_ObjectID_K1/1 -> AEBLatTargetObjectType/3(AEBLat_Target_ObjectID_K1)  "AEBLat_Target_ObjectID_K1"
  AEBLat_Target_ObjectType_K1/1 -> AEBLatTargetObjectType/4(AEBLat_Target_ObjectType_K1)  "AEBLat_Target_ObjectType_K1"

== system PubIfDecisionTOS_MDL/TOS_20201112/TOS_2012080320/TOS/AEB/TOS_AEBLatCro1105/AEBLat_Object_Condition/AEBLat_TargetCondition ==
  Object_ID : Inport  OutDataTypeStr=uint8  Partition=on  PartitionDimension=1  PartitionWidth=1  PartitionOffset=0
  PP_ObjFusType_FC_FR_Confirm : Inport  Port=2  Partition=on  PartitionDimension=1  PartitionWidth=1  PartitionOffset=0
  PP_ObjFusType_FR_Confirm : Inport  Port=3  Partition=on  PartitionDimension=1  PartitionWidth=1  PartitionOffset=0
  ObjectType : Inport  Port=4  Partition=on  PartitionDimension=1  PartitionWidth=1  PartitionOffset=0
  Object_Dx : Inport  Port=5  Partition=on  PartitionDimension=1  PartitionWidth=1  PartitionOffset=0
  Object_Dy : Inport  Port=6  Partition=on  PartitionDimension=1  PartitionWidth=1  PartitionOffset=0
  PP_ObjMovingDirSignalProcessing : Inport  Port=7  Partition=on  PartitionDimension=1  PartitionWidth=1  PartitionOffset=0
  Object_HeadingAngle : Inport  Port=8  Partition=on  PartitionDimension=1  PartitionWidth=1  PartitionOffset=0
  Object_VX : Inport  Port=9  Partition=on  PartitionDimension=1  PartitionWidth=1  PartitionOffset=0
  Object_VY : Inport  Port=10  Partition=on  PartitionDimension=1  PartitionWidth=1  PartitionOffset=0
  VIE_EgoVelocity : Inport  Port=11
  psiDtOpt : Inport  Port=12
  AEBLat_Target_ObjectID_K1 : Inport  Port=13
  Compare To Constant : simulink/Logic and Bit Operations/Compare To Constant  relop===  const=C_TOS_OFMObjIDInvilad_Val  OutDataTypeStr=boolean
      settings: AttributesFormatString=C_TOS_OFMObjIDInvilad_Val = 0
  For Each : ForEach  DisableCoverage=on
  If : If  IfExpression=u1 ~= 0
  Merge{,1..4} (5 alike) : Merge
  TOS_AEBLat_TargetsDx : Subsystem
  TOS_AEBLat_TargetsDxDefault : Subsystem  TreatAsAtomicUnit=on
  TOS_AEBLat_Targets_Dx : Outport  ConcatenationDimension=1
  AEBLat_TargetFusionType_observal : Outport  Port=2  ConcatenationDimension=1
  AEBLat_TargetObjectType_observal : Outport  Port=3  ConcatenationDimension=1
  AEBLat_TargetDXDY_observal : Outport  Port=4  ConcatenationDimension=1
  AEBLat_TargetMovDir_observal : Outport  Port=5  ConcatenationDimension=1
  wires:
  PP_ObjFusType_FC_FR_Confirm/1 -> TOS_AEBLat_TargetsDx/2(PP_ObjFusType_FC_FR_Confirm)
  PP_ObjFusType_FR_Confirm/1 -> TOS_AEBLat_TargetsDx/3(PP_ObjFusType_FR_Confirm)
  Object_VY/1 -> TOS_AEBLat_TargetsDx/10(Object_VY)
  VIE_EgoVelocity/1 -> TOS_AEBLat_TargetsDx/11(VIE_EgoVelocity)
  Object_VX/1 -> TOS_AEBLat_TargetsDx/9(Object_VX)
  PP_ObjMovingDirSignalProcessing/1 -> TOS_AEBLat_TargetsDx/7(PP_ObjMovingDirSignalProcessing)
  Object_HeadingAngle/1 -> TOS_AEBLat_TargetsDx/8(Object_HeadingAngle)
  ObjectType/1 -> TOS_AEBLat_TargetsDx/4(ObjectType)
  TOS_AEBLat_TargetsDxDefault/1(TOS_AEBLong_TargetsDx) -> Merge/1
  If/2 -> TOS_AEBLat_TargetsDx/Action
  If/1 -> TOS_AEBLat_TargetsDxDefault/Action
  Object_ID/1 -> Compare To Constant/1, [Object_ID]
  Compare To Constant/1 -> If/1
  TOS_AEBLat_TargetsDx/1(TOS_AEBLat_TargetsDx) -> Merge/2
  Object_Dy/1 -> TOS_AEBLat_TargetsDx/6(Object_Dy)
  Object_Dx/1 -> TOS_AEBLat_TargetsDx/5(Object_Dx)
  Merge/1 -> TOS_AEBLat_Targets_Dx/1
  TOS_AEBLat_TargetsDx/2(AEBLat_TargetFusionType_observal) -> Merge1/2
  TOS_AEBLat_TargetsDxDefault/2(AEBLong_TargetFusionType_observal) -> Merge1/1
  TOS_AEBLat_TargetsDxDefault/3(AEBLong_TargetObjectType_observal) -> Merge2/1
  TOS_AEBLat_TargetsDx/3(AEBLat_TargetObjectType_observal) -> Merge2/2
  TOS_AEBLat_TargetsDx/4(AEBLat_TargetDXDY_observal) -> Merge3/2
  TOS_AEBLat_TargetsDxDefault/4(AEBLong_TargetDXDY_observal) -> Merge3/1
  TOS_AEBLat_TargetsDxDefault/5(AEBLong_TargetMovDir_observal) -> Merge4/1
  TOS_AEBLat_TargetsDx/5(AEBLat_TargetMovDir_observal) -> Merge4/2
  Merge1/1 -> AEBLat_TargetFusionType_observal/1
  Merge2/1 -> AEBLat_TargetObjectType_observal/1
  Merge3/1 -> AEBLat_TargetDXDY_observal/1
  Merge4/1 -> AEBLat_TargetMovDir_observal/1
  [Object_ID] -> TOS_AEBLat_TargetsDx/1(Object_ID)  "Object_ID"
  AEBLat_Target_ObjectID_K1/1 -> TOS_AEBLat_TargetsDx/13(AEBLat_Target_ObjectID_K1)
  psiDtOpt/1 -> TOS_AEBLat_TargetsDx/12(psiDtOpt)

== system PubIfDecisionTOS_MDL/TOS_20201112/TOS_2012080320/TOS/AEB/TOS_AEBLatCro1105/AEBLat_Object_Condition2/AEBLat_TargetCondition ==
  Object_ID : Inport  OutDataTypeStr=uint8  Partition=on  PartitionDimension=1  PartitionWidth=1  PartitionOffset=0
  PP_ObjFusType_FC_FR_Confirm : Inport  Port=2  Partition=on  PartitionDimension=1  PartitionWidth=1  PartitionOffset=0
  PP_ObjFusType_FR_Confirm : Inport  Port=3  Partition=on  PartitionDimension=1  PartitionWidth=1  PartitionOffset=0
  ObjectType : Inport  Port=4  Partition=on  PartitionDimension=1  PartitionWidth=1  PartitionOffset=0
  Object_Dx : Inport  Port=5  Partition=on  PartitionDimension=1  PartitionWidth=1  PartitionOffset=0
  Object_Dy : Inport  Port=6  Partition=on  PartitionDimension=1  PartitionWidth=1  PartitionOffset=0
  PP_ObjMovingDirSignalProcessing : Inport  Port=7  Partition=on  PartitionDimension=1  PartitionWidth=1  PartitionOffset=0
  Object_HeadingAngle : Inport  Port=8  Partition=on  PartitionDimension=1  PartitionWidth=1  PartitionOffset=0
  Object_VX : Inport  Port=9  Partition=on  PartitionDimension=1  PartitionWidth=1  PartitionOffset=0
  Object_VY : Inport  Port=10  Partition=on  PartitionDimension=1  PartitionWidth=1  PartitionOffset=0
  VIE_EgoVelocity : Inport  Port=11
  psiDtOpt : Inport  Port=12
  AEBLat_Target_ObjectID_K1 : Inport  Port=13
  Compare To Constant : simulink/Logic and Bit Operations/Compare To Constant  relop===  const=C_TOS_OFMObjIDInvilad_Val  OutDataTypeStr=boolean
      settings: AttributesFormatString=C_TOS_OFMObjIDInvilad_Val = 0
  For Each : ForEach  DisableCoverage=on
  If : If  IfExpression=u1 ~= 0
  Merge{,1..4} (5 alike) : Merge
  TOS_AEBLat_TargetsDx : Subsystem
  TOS_AEBLat_TargetsDxDefault : Subsystem  TreatAsAtomicUnit=on
  TOS_AEBLat_Targets_Dx : Outport  ConcatenationDimension=1
  AEBLat_TargetFusionType_observal : Outport  Port=2  ConcatenationDimension=1
  AEBLat_TargetObjectType_observal : Outport  Port=3  ConcatenationDimension=1
  AEBLat_TargetDXDY_observal : Outport  Port=4  ConcatenationDimension=1
  AEBLat_TargetMovDir_observal : Outport  Port=5  ConcatenationDimension=1
  wires:
  PP_ObjFusType_FC_FR_Confirm/1 -> TOS_AEBLat_TargetsDx/2(PP_ObjFusType_FC_FR_Confirm)
  PP_ObjFusType_FR_Confirm/1 -> TOS_AEBLat_TargetsDx/3(PP_ObjFusType_FR_Confirm)
  Object_VY/1 -> TOS_AEBLat_TargetsDx/10(Object_VY)
  VIE_EgoVelocity/1 -> TOS_AEBLat_TargetsDx/11(VIE_EgoVelocity)
  Object_VX/1 -> TOS_AEBLat_TargetsDx/9(Object_VX)
  PP_ObjMovingDirSignalProcessing/1 -> TOS_AEBLat_TargetsDx/7(PP_ObjMovingDirSignalProcessing)
  Object_HeadingAngle/1 -> TOS_AEBLat_TargetsDx/8(Object_HeadingAngle)
  ObjectType/1 -> TOS_AEBLat_TargetsDx/4(ObjectType)
  TOS_AEBLat_TargetsDxDefault/1(TOS_AEBLong_TargetsDx) -> Merge/1
  If/2 -> TOS_AEBLat_TargetsDx/Action
  If/1 -> TOS_AEBLat_TargetsDxDefault/Action
  Object_ID/1 -> Compare To Constant/1, [Object_ID]
  Compare To Constant/1 -> If/1
  TOS_AEBLat_TargetsDx/1(TOS_AEBLat_TargetsDx) -> Merge/2
  Object_Dy/1 -> TOS_AEBLat_TargetsDx/6(Object_Dy)
  Object_Dx/1 -> TOS_AEBLat_TargetsDx/5(Object_Dx)
  Merge/1 -> TOS_AEBLat_Targets_Dx/1
  TOS_AEBLat_TargetsDx/2(AEBLat_TargetFusionType_observal) -> Merge1/2
  TOS_AEBLat_TargetsDxDefault/2(AEBLong_TargetFusionType_observal) -> Merge1/1
  TOS_AEBLat_TargetsDxDefault/3(AEBLong_TargetObjectType_observal) -> Merge2/1
  TOS_AEBLat_TargetsDx/3(AEBLat_TargetObjectType_observal) -> Merge2/2
  TOS_AEBLat_TargetsDx/4(AEBLat_TargetDXDY_observal) -> Merge3/2
  TOS_AEBLat_TargetsDxDefault/4(AEBLong_TargetDXDY_observal) -> Merge3/1
  TOS_AEBLat_TargetsDxDefault/5(AEBLong_TargetMovDir_observal) -> Merge4/1
  TOS_AEBLat_TargetsDx/5(AEBLat_TargetMovDir_observal) -> Merge4/2
  Merge1/1 -> AEBLat_TargetFusionType_observal/1
  Merge2/1 -> AEBLat_TargetObjectType_observal/1
  Merge3/1 -> AEBLat_TargetDXDY_observal/1
  Merge4/1 -> AEBLat_TargetMovDir_observal/1
  [Object_ID] -> TOS_AEBLat_TargetsDx/1(Object_ID)  "Object_ID"
  AEBLat_Target_ObjectID_K1/1 -> TOS_AEBLat_TargetsDx/13(AEBLat_Target_ObjectID_K1)
  psiDtOpt/1 -> TOS_AEBLat_TargetsDx/12(psiDtOpt)

== system PubIfDecisionTOS_MDL/TOS_20201112/TOS_2012080320/TOS/AEB/TOS_AEBLatCro_20201208/AEBLatTrgInfor/AEBLatTargetObjectType ==
  OFM_SignalVerification : Inport
  AEBLat_Target_ObjectID_K1 : Inport  Port=2
  AEBLat_Target_ObjectType_K1 : Inport  Port=3
  TOS_AEBLatTrg_Index : Inport  Port=4  OutDataTypeStr=uint8  Partition=on  PartitionDimension=1  PartitionWidth=1  PartitionOffset=0
  AEBLatTargetObjectType : Subsystem  TreatAsAtomicUnit=on
  AEBLatTargetObjectTypeDefault : Subsystem  TreatAsAtomicUnit=on
  Compare To Constant1 : simulink/Logic and Bit Operations/Compare To Constant  relop===  const=C_TOS_OFMObjIDInvilad_Val  OutDataTypeStr=boolean
      settings: AttributesFormatString=C_TOS_OFMObjIDInvilad_Val = 0
  For Each : ForEach  DisableCoverage=on
  If : If  IfExpression=u1
  Merge : Merge
  TOS_AEBLatTargetObjectType : Outport  ConcatenationDimension=1
  wires:
  Merge/1 -> TOS_AEBLatTargetObjectType/1
  AEBLatTargetObjectTypeDefault/1(TOS_AEBLatTargetObjectType) -> Merge/1
  AEBLatTargetObjectType/1(AEBLat_TargetObjectType) -> Merge/2
  If/2 -> AEBLatTargetObjectType/Action
  If/1 -> AEBLatTargetObjectTypeDefault/Action
  OFM_SignalVerification/1 -> AEBLatTargetObjectType/2(OFM_SignalVerification)
  Compare To Constant1/1 -> If/1
  TOS_AEBLatTrg_Index/1 -> AEBLatTargetObjectType/1(TOS_AEBLatTrg_Index), Compare To Constant1/1
  AEBLat_Target_ObjectID_K1/1 -> AEBLatTargetObjectType/3(AEBLat_Target_ObjectID_K1)  "AEBLat_Target_ObjectID_K1"
  AEBLat_Target_ObjectType_K1/1 -> AEBLatTargetObjectType/4(AEBLat_Target_ObjectType_K1)  "AEBLat_Target_ObjectType_K1"
